simulink model "PickAndPlace_Hardware"  (R2024b)
settings: Solver=ode2  StartTime=0.0  StopTime=inf  FixedStep=0.005  RelTol=1e-3  EnableMultiTasking=on
InitFcn:
  | qarmRigidBodyTree = importrobot('Resources/qarm/urdf/QARM.urdf');
  | qarmRigidBodyTree.Bodies{1,3}.Joint.PositionLimits(1) = -pi/4;
  | show(qarmRigidBodyTree);
model workspace (MAT data in the model file):
  Sig = Simulink.Signal
  Sig.Dimensions = -1
  Sig.DimensionsMode = 'auto'
  Sig.Complexity = 'auto'
  Sig.SampleTime = -1
  Sig.SamplingMode = 'auto'
  Sig.DataType = 'auto'
undefined symbols (not defined in the file or in its folder): EFFECTOR, END, HIL, Levenberg, Marquardt
libraries: quarc_library x7, robotmaniplib x2
settings Model: ExtModeTrigDuration=10000  Creator=mbohra  LastModifiedBy=tongc
settings SolverCC: AlgebraicLoopSolver=TrustRegion  PositivePriorityOrder=on
settings DebuggingCC: UnconnectedInputMsg=warning  UnconnectedOutputMsg=warning  UnconnectedLineMsg=warning
settings ModelReferenceCC: EnableRefExpFcnMdlSchedulingChecks=on
settings SFSimCC: CustomCodeUndefinedFunction=UseInterfaceOnly
settings RTWCC: Description=QUARC Win64 Target Using Toolchain  SystemTargetFile=quarc_win64.tlc  TemplateMakefile=quarc_default_tmf  Toolchain=QUARC win64 | nmake (64-bit Windows)  BuildConfiguration=Faster Runs  GPUComputeCapability=3.5  DLArmComputeVersion=19.05
settings STFCustomTargetCC: TargetLangStandard=C99 (ISO)  ConcurrentExecutionCompliant=on  GRTInterface=on  UseToolchainInfoCompliant=on  SystemTargetFile=quarc_win64.tlc
settings GRTTargetCC: ParMdlRefBuildCompliant=off  CompOptLevelCompliant=off  CombineOutputUpdateFcns=off  MatFileLogging=off  CPPClassGenCompliant=off  GRTInterface=on  ExtMode=on  ExtModeMexFile=quarc_comm

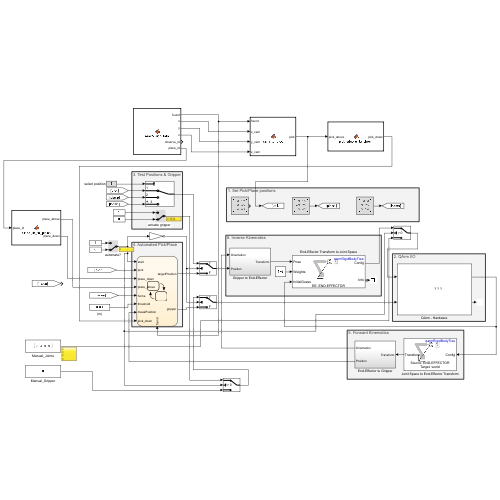
[thumbnail: Simulink's stored preview of the top-level diagram]
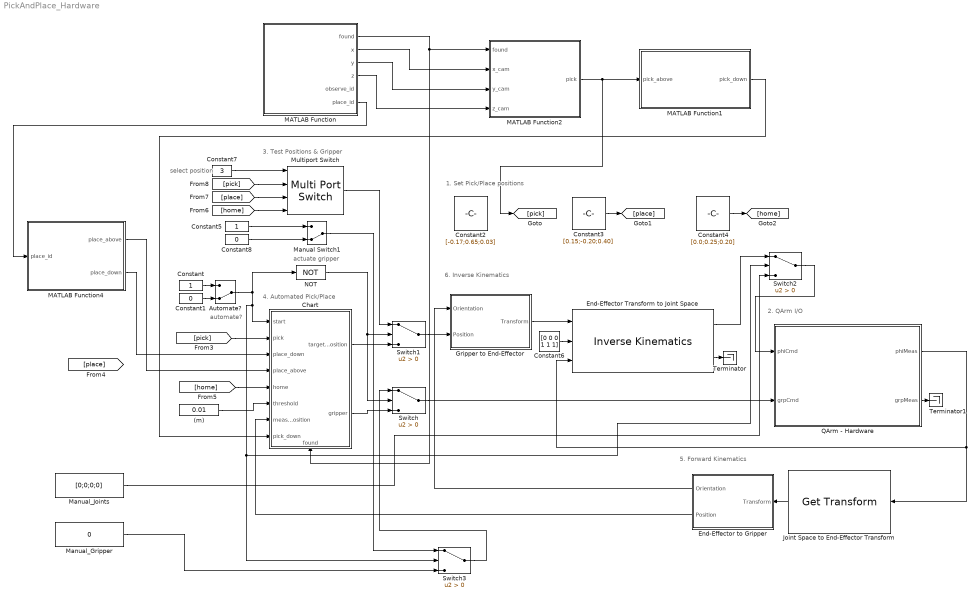
== system PickAndPlace_Hardware ==
  note: 2. QArm I/O
  note: 6. Inverse Kinematics
  note: 1. Set Pick/Place positions
  note: 3. Test Positions & Gripper
  note: 4. Automated Pick/Place
  note: select position
  note: 5. Forward Kinematics
  note: actuate gripper
  note: automate?
  (m) : Constant  Value=0.01
  Automate? : ManualSwitch  CurrentSetting=0
  Chart : Stateflow chart  TreatAsAtomicUnit=on
      settings: PortSchema="{\"entries\":[{\"content\":{\"sides\":[{\"content\":{\"connectorIds\":[\"In2\",\"In5\",\"In3\",\"In4\",\"In6\",\"In7\",\"In8\",\"In9\"]},\"type\":\"ConnectorPlacement.EquallySpacedRectSide\",\"uuid\":\"2311fb17-ea66-418d-9fcf-b7200b53fcca\"},{\"content\":{\"connectorIds\":[\"Out1\",\"Out2\"],\"side\":\"RIGHT\"},\"type\":\"ConnectorPlacement.EquallySpacedRectSide\",\"uuid\":\"022a4bb9-2bc3-44ee-b083-520032a85134\"},{\"content\":{\"side\":\"TOP\"},\"type\":\"ConnectorPlacement.EquallySpacedRectSide\",\"uuid\":\"39e1e844-d468-4b0c-88d8-3a69ec67319a\"},{\"content\":{\"connectorIds\":[\"In1\"],\"side\":\"BOTTOM\"},\"type\":\"ConnectorPlacement.EquallySpacedRectSide\",\"uuid\":\"44731073-2af9-4c99-b878-93e346118474\"}]},\"type\":\"ConnectorPlacement.EquallySpacedConnector\",\"uuid\":\"fe0d806d-7322-4085-bccb-c8355c39d6a3\"}],\"packageUris\":[\"http://schema.mathworks.com/mf0/Connector/R2020b\"],\"version\":\"1.0\"}"
  Constant : Constant
  Constant1 : Constant  Value=0
  Constant2 : Constant  Value=[-0.17;0.65;0.03]  VectorParams1D=off
  Constant3 : Constant  Value=[0.15;-0.20;0.40]  VectorParams1D=off
  Constant4 : Constant  Value=[0.0;0.25;0.20]  VectorParams1D=off
  Constant5 : Constant
  Constant6 : Constant  Value=[0 0 0 1 1 1]
  Constant7 : Constant  Value=3
  Constant8 : Constant  Value=0
  End-Effector Transform to Joint Space : robotmaniplib/Inverse Kinematics  RigidBodyTree=qarmRigidBodyTree  EndEffector=END-EFFECTOR  ShowInfo=on  SolverName=Levenberg-Marquardt  EnforceJointLimits=on  MaxIterations=2  MaxTime=qc_get_step_size  GradientTolerance=1e-4  SolutionTolerance=1e-3  StepTolerance=1e-3  ErrorChangeTolerance=1e-6  UseErrorDamping=on  DampingBias=0.0025  SimulateUsing=Code generation
  End-Effector to Gripper : Subsystem
  Gripper to End-Effector : Subsystem
  Joint Space to End-Effector Transform : robotmaniplib/Get Transform  RigidBodyTree=qarmRigidBodyTree  SourceBody=END-EFFECTOR  TargetBody=world  SimulateUsing=Interpreted execution
  MATLAB Function : MATLAB Function  TreatAsAtomicUnit=on
  MATLAB Function1 : MATLAB Function  TreatAsAtomicUnit=on
  MATLAB Function2 : MATLAB Function  TreatAsAtomicUnit=on
  MATLAB Function4 : MATLAB Function  TreatAsAtomicUnit=on
  Manual Switch1 : ManualSwitch  CurrentSetting=0
  Manual_Gripper : Constant  Value=0
  Manual_Joints : Constant  Value=[0;0;0;0]
  Multiport Switch : MultiPortSwitch  SaturateOnIntegerOverflow=off  InputSameDT=off
  NOT : Logic  Operator=NOT  IconShape=distinctive  AllPortsSameDT=off  OutDataTypeStr=boolean
  QArm - Hardware : Subsystem
      mask Display:
      | image('Resources/QArm.png')
      | port_label('input', 1, 'phiCmd');
      | port_label('input', 2, 'grpCmd');
      | port_label('output', 1, 'phiMeas');
      | port_label('output', 2, 'grpMeas');
  Switch{,1..3} (4 alike) : Switch  Criteria=u2 > Threshold  SaturateOnIntegerOverflow=off  InputSameDT=off
  Terminator : Terminator
  Terminator1 : Terminator
  wires:
  Constant/1 -> Automate?/1
  Constant1/1 -> Automate?/2
  Automate?/1 -> Switch3/2, Switch2/2, Chart/2(start), NOT/1
  [pick] -> Chart/5(pick)
  [home] -> Chart/6(home)
  Constant6/1 -> End-Effector Transform to Joint Space/2
  Chart/2(gripper) -> Switch/3
  Constant7/1 -> Multiport Switch/1
  Chart/1(targetPosition) -> Switch1/3
  Multiport Switch/1 -> Switch1/1
  Constant5/1 -> Manual Switch1/1
  Constant8/1 -> Manual Switch1/2
  Constant4/1 -> [home]
  [home] -> Multiport Switch/4
  [place] -> Multiport Switch/3
  [pick] -> Multiport Switch/2
  End-Effector to Gripper/2(Position) -> Chart/8(measPosition)
  (m)/1 -> Chart/7(threshold)
  Switch1/1 -> Gripper to End-Effector/2(Position)
  End-Effector to Gripper/1(Orientation) -> Gripper to End-Effector/1(Orientation)
  Gripper to End-Effector/1(Transform) -> End-Effector Transform to Joint Space/1
  End-Effector Transform to Joint Space/2 -> Terminator/1
  Joint Space to End-Effector Transform/1 -> End-Effector to Gripper/1(Transform)
  NOT/1 -> Switch1/2, Switch/2
  QArm - Hardware/1(phiMeas) -> End-Effector Transform to Joint Space/3, Joint Space to End-Effector Transform/1
  Switch/1 -> QArm - Hardware/2(grpCmd)
  QArm - Hardware/2(grpMeas) -> Terminator1/1
  MATLAB Function/1(found) -> Chart/1(found), MATLAB Function2/1(found)
  MATLAB Function/2(x) -> MATLAB Function2/2(x_cam)
  MATLAB Function/3(y) -> MATLAB Function2/3(y_cam)
  MATLAB Function/4(z) -> MATLAB Function2/4(z_cam)
  MATLAB Function2/1(pick) -> [pick], MATLAB Function1/1(pick_above)
  MATLAB Function1/1(pick_down) -> Chart/9(pick_down)
  Constant3/1 -> [place]
  MATLAB Function/6(place_id) -> MATLAB Function4/1(place_id)
  MATLAB Function4/2(place_down) -> Chart/3(place_down)
  MATLAB Function4/1(place_above) -> Chart/4(place_above)
  End-Effector Transform to Joint Space/1 -> Switch2/1
  Switch2/1 -> QArm - Hardware/1(phiCmd)
  Manual_Joints/1 -> Switch2/3
  Manual Switch1/1 -> Switch3/1
  Switch3/1 -> Switch/1
  Manual_Gripper/1 -> Switch3/3

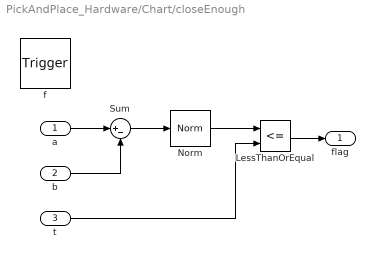
== system PickAndPlace_Hardware/Chart/closeEnough ==
  a : Inport  OutDataTypeStr=double  PortDimensions=[3,1]
  b : Inport  Port=2  OutDataTypeStr=double  PortDimensions=[3,1]
  t : Inport  Port=3  OutDataTypeStr=double  PortDimensions=[1]
  f : TriggerPort  TriggerType=function-call  VariantControl=(inherit)
      settings: CopyFcn=Stateflow.SLINSF.SimulinkMan.removeBlockPreDeleteFcn  PreDeleteFcn=Stateflow.SLINSF.SimulinkMan.unsafePredeleteFcn
  LessThanOrEqual : RelationalOperator  Operator=<=  OutDataTypeStr=boolean  RndMeth=Simplest  InputSameDT=off
  Norm : quarc_library/Math Operations/Vectors/Norm
      settings: SourceProductName=QUARC Targets
  Sum : Sum  Inputs=|+-
  flag : Outport  VectorParamsAs1DForOutWhenUnconnected=off
  wires:
  a/1 -> Sum/1
  b/1 -> Sum/2
  Sum/1 -> Norm/1
  Norm/1 -> LessThanOrEqual/1
  t/1 -> LessThanOrEqual/2
  LessThanOrEqual/1 -> flag/1

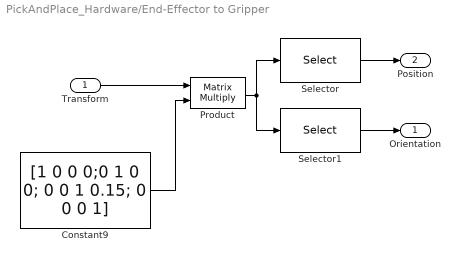
== system PickAndPlace_Hardware/End-Effector to Gripper ==
  Transform : Inport
  Constant9 : Constant  Value=[1 0 0 0;0 1 0 0; 0 0 1 0.15; 0 0 0 1]  VectorParams1D=off
  Product : Product  Multiplication=Matrix(*)
  Selector : Selector  NumberOfDimensions=2  InputPortWidth=3  IndexOptions=Index vector (dialog),Index vector (dialog)  Indices=[1:3],4  OutputSizes=1,1
  Selector1 : Selector  NumberOfDimensions=2  InputPortWidth=3  IndexOptions=Index vector (dialog),Index vector (dialog)  Indices=[1:3],[1:3]  OutputSizes=1,1
  Orientation : Outport
  Position : Outport  Port=2
  wires:
  Transform/1 -> Product/1
  Product/1 -> Selector/1, Selector1/1
  Selector/1 -> Position/1
  Constant9/1 -> Product/2
  Selector1/1 -> Orientation/1

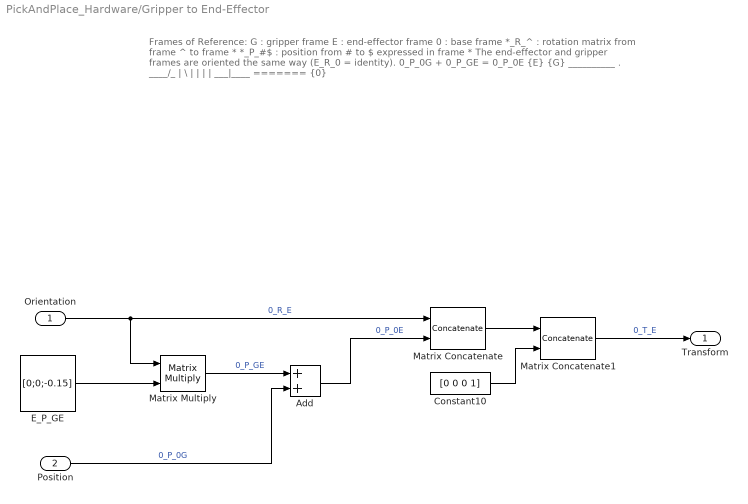
== system PickAndPlace_Hardware/Gripper to End-Effector ==
  note: Frames of Reference:
      |
      | G : gripper frame
      | E : end-effector frame
      | 0 : base frame
      | *_R_^ : rotation matrix from frame ^ to frame *
      | *_P_#$ : position from # to $ expressed in frame *
      |
      | The end-effector and gripper frames are oriented the same way (E_R_0 = identity).
      | 0_P_0G + 0_P_GE = 0_P_0E
      |
      | {E} {G}
      | __________ . ____/_
      | | \
      | |
      | |
      | |
      | |
      | ___|____
      | =======
      | {0}
  Orientation : Inport
  Position : Inport  Port=2
  Add : Sum
  Constant10 : Constant  Value=[0 0 0 1]  VectorParams1D=off
  E_P_GE : Constant  Value=[0;0;-0.15]  VectorParams1D=off
  Matrix Concatenate : Concatenate  Mode=Multidimensional array  ConcatenateDimension=2
  Matrix Concatenate1 : Concatenate  Mode=Multidimensional array
  Matrix Multiply : Product  Multiplication=Matrix(*)
  Transform : Outport
  wires:
  Matrix Concatenate/1 -> Matrix Concatenate1/1
  Orientation/1 -> Matrix Concatenate/1, Matrix Multiply/1  "0_R_E"
  Constant10/1 -> Matrix Concatenate1/2
  Matrix Concatenate1/1 -> Transform/1  "0_T_E"
  Matrix Multiply/1 -> Add/1  "0_P_GE"
  Position/1 -> Add/2  "0_P_0G"
  E_P_GE/1 -> Matrix Multiply/2
  Add/1 -> Matrix Concatenate/2  "0_P_0E"

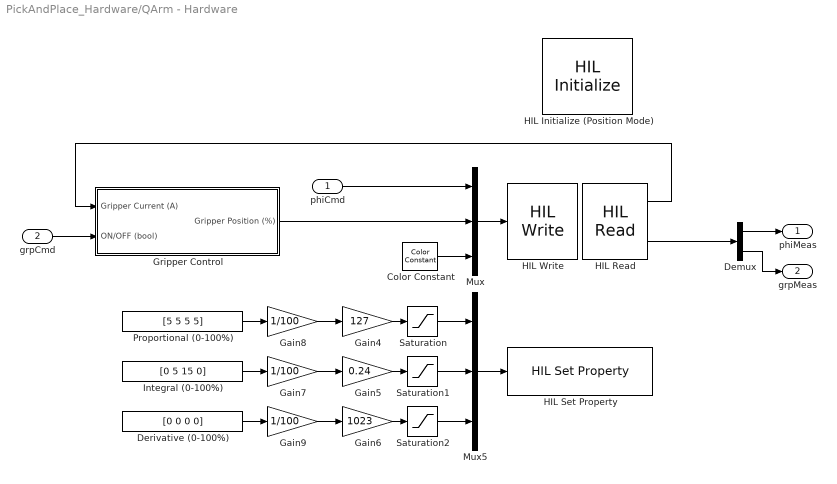
== system PickAndPlace_Hardware/QArm - Hardware ==
  phiCmd : Inport
  grpCmd : Inport  Port=2
  Color Constant : quarc_library/Sources/Signals/Color Constant  color=[0 1 0]
      settings: SourceProductName=QUARC Targets
  Demux : Demux  Outputs=[4 1]
  Derivative (0-100%) : Constant  Value=[0 0 0 0]
  Gain4 : Gain  Gain=127
  Gain5 : Gain  Gain=0.24
  Gain6 : Gain  Gain=1023
  Gain7 : Gain  Gain=1/100
  Gain8 : Gain  Gain=1/100
  Gain9 : Gain  Gain=1/100
  Gripper Control : Subsystem
  HIL Initialize (Position Mode) : quarc_library/Data Acquisition/Generic/Configuration/HIL Initialize  object_name=HIL-1  board_type=qarm_usb  board_number=0  board_options=j0_mode=0;j1_mode=0;j2_mode=0;j3_mode=0;gripper_mode=0;j0_profile_config=0;j0_profile_velocity=1.5708;j0_profile_acceleration=1.5708;j1_profile_config=0;j1_profile_velocity=1.5708;j1_profile_acceleration=1.5708;j2_profile_config=0;j2_profile_velocity=1.5708;j2_profile_acceleration=1.5708;j3_profile_config=0;j3_profile_velocity=1.5708;j3_profile_acceleration=1.5708;  exclusive=off  active=on  hardware_clocks=[0]  clock_modes=[]  initial_clock_frequencies=[]  set_clock_params_at_start=off  set_clock_params_at_switch_in=off  set_clock_frequencies_at_start=off  set_clock_frequencies_at_switch_in=off  analog_input_channels=[5:9]  analog_input_configurations=[]  analog_input_maximums=[]  analog_input_minimums=[]  set_analog_input_params_at_start=off  set_analog_input_params_at_switch_in=off  analog_output_channels=[]  analog_output_maximums=inf  analog_output_minimums=-inf  initial_analog_outputs=[0]  final_analog_outputs=[0]  watchdog_analog_outputs=[]  set_analog_output_params_at_start=off  set_analog_output_params_at_switch_in=off  set_analog_outputs_at_start=off  set_analog_outputs_at_switch_in=off  set_analog_outputs_at_terminate=off  set_analog_outputs_at_switch_out=off  set_analog_outputs_on_watchdog=off  digital_input_channels=[]  digital_output_channels=[]  digital_output_configuration=[]  initial_digital_outputs=[0]  final_digital_outputs=[0]  watchdog_digital_outputs=[0]  set_digital_output_params_at_start=off  set_digital_output_params_at_switch_in=off  set_digital_outputs_at_start=off  set_digital_outputs_at_switch_in=off  set_digital_outputs_at_terminate=off  set_digital_outputs_at_switch_out=off  set_digital_outputs_on_watchdog=off  encoder_channels=[]  quadrature=[]  encoder_filter_frequency=[]  initial_encoder_counts=[]  set_encoder_params_at_start=off  set_encoder_params_at_switch_in=off  set_encoder_counts_at_start=off  set_encoder_counts_at_switch_in=off  pwm_channels=[]  pwm_modes=[]  pwm_frequency=[]  pwm_configuration=[]  pwm_alignment=[]  pwm_polarity=[]  pwm_leading_deadband=[]  pwm_trailing_deadband=[]  initial_pwm_outputs=[]  final_pwm_outputs=[]  watchdog_pwm_outputs=[]  set_pwm_params_at_start=off  set_pwm_params_at_switch_in=off  set_pwm_outputs_at_start=off  set_pwm_outputs_at_switch_in=off  set_pwm_outputs_at_terminate=off  set_pwm_outputs_at_switch_out=off  set_pwm_outputs_on_watchdog=off  other_output_channels=[1000:1004 11000:11003 11005:11007]  initial_other_outputs=[zeros(1,9), ones(1,3)]  final_other_outputs=[zeros(1,9), ones(1,3)]  watchdog_other_outputs=zeros(1,12)  set_other_outputs_at_start=off  set_other_outputs_at_switch_in=off  set_other_outputs_at_terminate=on  set_other_outputs_at_switch_out=off  set_other_outputs_on_watchdog=off
      settings: AttributesFormatString=%<object_name> (%<board_type>-%<board_number>)
  HIL Read : quarc_library/Data Acquisition/Generic/Immediate I//O/HIL Read  object_name=HIL-1  analog_channels=[9]  encoder_channels=[]  digital_channels=[]  other_channels=[1000:1004]  sample_time=qc_get_step_size  active=on  vector_output=on  data_type_mode=Inherit via back propagation  encoder_data_type=double  digital_data_type=boolean
  HIL Set Property : quarc_library/Data Acquisition/Generic/Configuration/HIL Set Property  object_name=HIL-1  property_type=2  property_codes=[128:131, 133:136, 138:141]  property_source=2  property_value_num=0  set_at_start=on  sample_time=-1  active=on
      settings: AttributesFormatString=(%<object_name>)  SourceProductName=QUARC Targets
  HIL Write : quarc_library/Data Acquisition/Generic/Immediate I//O/HIL Write  object_name=HIL-1  analog_channels=[]  pwm_channels=[]  digital_channels=[]  other_channels=[1000:1004 11005:11007]  sample_time=-1  active=on  vector_input=on
  Integral (0-100%) : Constant  Value=[0 5 15 0]
  Mux : Mux  Inputs=3
  Mux5 : Mux  Inputs=3
  Proportional (0-100%) : Constant  Value=[5 5 5 5]
  Saturation : Saturate  UpperLimit=127  LowerLimit=0
  Saturation1 : Saturate  UpperLimit=0.24  LowerLimit=0
  Saturation2 : Saturate  UpperLimit=1023  LowerLimit=0
  phiMeas : Outport
  grpMeas : Outport  Port=2
  wires:
  Mux/1 -> HIL Write/1
  Color Constant/1 -> Mux/3
  phiCmd/1 -> Mux/1
  Demux/1 -> phiMeas/1
  Demux/2 -> grpMeas/1
  Integral (0-100%)/1 -> Gain7/1
  Mux5/1 -> HIL Set Property/1
  Gain9/1 -> Gain6/1
  Gain6/1 -> Saturation2/1
  Saturation2/1 -> Mux5/3
  Saturation/1 -> Mux5/1
  Gain5/1 -> Saturation1/1
  Gain8/1 -> Gain4/1
  Proportional (0-100%)/1 -> Gain8/1
  Gain7/1 -> Gain5/1
  Saturation1/1 -> Mux5/2
  Gain4/1 -> Saturation/1
  Derivative (0-100%)/1 -> Gain9/1
  Gripper Control/1(Gripper Position (%)) -> Mux/2
  grpCmd/1 -> Gripper Control/2(ON/OFF (bool))
  HIL Read/2 -> Demux/1
  HIL Read/1 -> Gripper Control/1(Gripper Current (A))

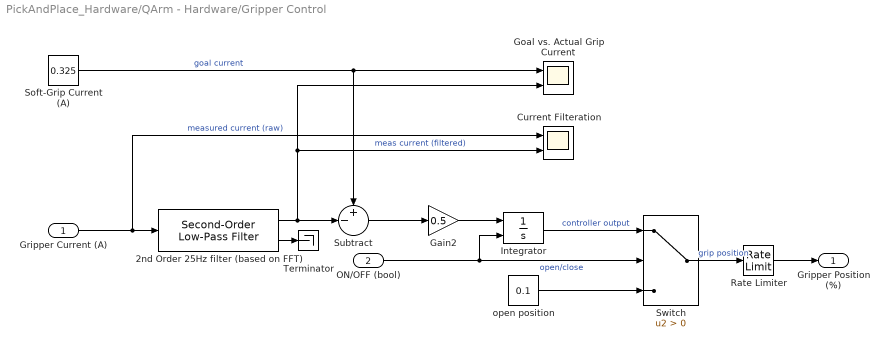
== system PickAndPlace_Hardware/QArm - Hardware/Gripper Control ==
  Gripper Current (A) : Inport
  ON/OFF (bool) : Inport  Port=2
  2nd Order 25Hz filter (based on FFT) : quarc_library/Continuous/Second-Order Low-Pass Filter  params_source=Internal (dialog parameters)  input_width=25*2*pi  input_zeta=1  input_init=0
  Current Filteration : Scope  NumInputPorts=2
  Gain2 : Gain  Gain=0.5
  Goal vs. Actual Grip Current : Scope  NumInputPorts=2
  Integrator : Integrator  ExternalReset=either  InitialCondition=0.1  LimitOutput=on  UpperSaturationLimit=0.9  LowerSaturationLimit=0.1
  Rate Limiter : RateLimiter  SampleTimeMode=inherited
  Soft-Grip Current (A) : Constant  Value=0.325
  Subtract : Sum  Inputs=+-|
  Switch : Switch  Criteria=u2 > Threshold  SaturateOnIntegerOverflow=off  InputSameDT=off
  Terminator : Terminator
  open position : Constant  Value=0.1
  Gripper Position (%) : Outport  VectorParamsAs1DForOutWhenUnconnected=off
  wires:
  Gripper Current (A)/1 -> 2nd Order 25Hz filter (based on FFT)/1, Current Filteration/1  "measured current (raw)"
  ON/OFF (bool)/1 -> Switch/2, Integrator/2  "open/close"
  open position/1 -> Switch/3
  Switch/1 -> Rate Limiter/1  "grip position"
  Soft-Grip Current (A)/1 -> Subtract/1, Goal vs. Actual Grip Current/1  "goal current"
  2nd Order 25Hz filter (based on FFT)/1 -> Subtract/2, Current Filteration/2, Goal vs. Actual Grip Current/2  "meas current (filtered)"
  Subtract/1 -> Gain2/1
  Integrator/1 -> Switch/1  "controller output"
  Gain2/1 -> Integrator/1
  2nd Order 25Hz filter (based on FFT)/2 -> Terminator/1
  Rate Limiter/1 -> Gripper Position (%)/1

== matlab function PickAndPlace_Hardware/MATLAB Function1 ==
  data: pick_above input; pick_down output
function pick_down = pick_above_to_down(pick_above)

pick_down = pick_above;

% 只改 z，向下探
pick_down(3) = 0.02;

== matlab function PickAndPlace_Hardware/MATLAB Function ==
  data: found output; x output; y output; z output; observe_id output; place_id output
function [found, x, y, z, observe_id, place_id] = readVisionData()

coder.extrinsic('read_vision_result');

found = false;
x = 0;
y = 0;
z = 0;
observe_id = 0;
place_id = 0;

[found, x, y, z, observe_id, place_id] = read_vision_result();

end

== stateflow chart PickAndPlace_Hardware/Chart ==
  state Wait
    gripper=0;
    targetPosition=home;
  state DetectGoHome
    targetPosition = home;
    gripper = 0;
    flag = closeEnough(measPosition, targetPosition, threshold);
  state flag = closeEnough(a,b,t) [function]
  state GotoPickDown
    targetPosition = locked_pick_down;
    flag = closeEnough(measPosition, targetPosition, threshold);
  state DetectStable
    during:
    targetPosition = home;
    gripper = 0;
    exit:
    if found == 1
    locked_pick = pick;
    locked_pick_down = pick_down;
    locked_place_above = place_above;
    locked_place_down = place_down;
    end
  state GotoPick
    targetPosition = locked_pick;
    flag = closeEnough(measPosition, targetPosition, threshold);
  state CloseGripper
    gripper=1;
  state GotoHome
    targetPosition=home;
    flag = closeEnough(measPosition, targetPosition, threshold);
  state GotoHomeUp
    targetPosition = [0; 0.25; 0.45];
    flag = closeEnough(measPosition, targetPosition, threshold);
  state GotoPlaceAbove
    targetPosition = locked_place_above;
    flag = closeEnough(measPosition, targetPosition, threshold);
  state GotoPlaceAboveBack
    targetPosition = locked_place_above;
    flag = closeEnough(measPosition, targetPosition, threshold);
  state OpenGripper
    gripper=0;
  state GotoPlaceDown
    targetPosition = locked_place_down;
    flag = closeEnough(measPosition, targetPosition, threshold);
  (default) -> Wait
  Wait -> DetectGoHome : [start && after(10,sec)]
  DetectGoHome -> DetectStable : [flag]
  GotoPickDown -> CloseGripper : [after(10,sec) && flag]
  GotoHome -> DetectGoHome [order 2] : [after(10,sec) && flag]
  GotoPick -> GotoPickDown [order 1] : [gripper==0 && after(10,sec) && flag]
  DetectStable -> GotoPick : [after(25,sec) && found == 1]
  CloseGripper -> GotoPick : [gripper && after(10,sec)]
  GotoPick -> GotoHome [order 2] : [gripper==1 && after(10,sec)]
  GotoHomeUp -> GotoHome : [after(15,sec) && flag]
  GotoHome -> GotoPlaceAbove [order 1] : [gripper && after(10,sec) && flag]
  GotoPlaceAboveBack -> GotoHomeUp : [after(10,sec) && flag]
  GotoPlaceAbove -> GotoPlaceDown : [after(10,sec) && flag]
  OpenGripper -> GotoPlaceAboveBack : [after(5,sec)]
  GotoPlaceDown -> OpenGripper : [after(10,sec) && flag]
  data: a function_input double size=[3,1]; b function_input double size=[3,1]; flag function_output; t function_input double size=[1]; found input; start input; place_down input; place_above input; pick input size=[3,1]; targetPosition output size=[3,1]; gripper output size=[1]; home input double size=[3,1]; threshold input; measPosition input double size=[3,1]; flag local; pick_down input; locked_pick local double size=[3,1]; locked_pick_down local double size=[3,1]; locked_place local double size=[3,1]; locked_place_above local double size=[3,1] =[0.05; 0.45; 0.50]; locked_place_down local double size=[3,1] =[0.05; 0.45; 0.25]

== matlab function PickAndPlace_Hardware/MATLAB Function2 ==
  data: found input; pick output; x_cam input; y_cam input; z_cam input
function pick = cam_to_pick(found, x_cam, y_cam, z_cam)

% 默认安全点
pick = [0.00; 0.45; 0.10];

if found == 1

    % ===== 坐标转换（核心）=====
    x_robot = 0.9912*x_cam + 0.3656*y_cam + 0.4169*z_cam - 0.2121;
    y_robot = -0.0050*x_cam - 1.0058*y_cam + 0.2250*z_cam + 0.3782;

    % ===== 高度策略 =====
    z_robot = 0.15;   % 先到上方

    % ===== 限幅（防飞）=====
    x_robot = min(max(x_robot, -0.18), 0.18);
    y_robot = min(max(y_robot,  0.35), 0.65);
    z_robot = min(max(z_robot,  0.08), 0.15);

    pick = [x_robot; y_robot; z_robot];

end

== matlab function PickAndPlace_Hardware/MATLAB Function4 ==
  data: place_id input; place_above output; place_down output
function [place_above, place_down] = place_id_to_place(place_id)

% 统一放置上方安全点
place_above = [0.05; -0.30; 0.50];

% 默认下降点
place_down = [0.05; -0.30; 0.25];

if place_id == 1        % 香蕉
    place_down = [0.05; -0.30; 0.25];

elseif place_id == 2    % 草莓
    place_down = [-0.07; -0.30; 0.25];

elseif place_id == 3    % 番茄
    place_down = [-0.23; -0.30; 0.25];
end

end
